simulink model "gm_soc_dvbs2_fpga"  (R2025b)
settings: Solver=VariableStepAuto  StartTime=0.0  StopTime=10.0  RelTol=1e-3
InitFcn:
  | soc_dvbs2_init;
undefined symbols (not defined in the file or in its folder): Add, coefficientsLog, coefficientsSqrt1, coefficientsSqrt2, dataBits, Deinterleaver, designMultirateFIR, noisePow, Shift, Short, soc_dvbs2_designFIRFilter, soc_dvbs2_txPacketBits, syncWord, txDataOut, txFiltCoeff, XData
libraries: simulink x304, hdlsllib x265, dspsigops x15, dsphdlfiltering2 x8, hdlmdlgenlib x6, dsphdlsigops2 x5, commseqgen3 x5, dsphdlmathfun2 x3, hwlogicconnlib x2, whdledac x2, commhdlcrc x2, whdlutilities x1
(part 15 of 36)

== system gm_soc_dvbs2_fpga/DVBS2/DVBS2 TxRx/Channel/AWGN Generator/Unit Variance Gaussian Noise/TausUniformRandGen/TausURNG2 ==
  note: S1
  note: S1
  note: S0
  Bit Shift : hdlsllib/Logic and Bit Operations/Bit Shift  mode=Shift Left Logical  N=double(13)
  Bit Shift1 : hdlsllib/Logic and Bit Operations/Bit Shift  mode=Shift Right Logical  N=double(19)
  Bit Shift2 : hdlsllib/Logic and Bit Operations/Bit Shift  mode=Shift Left Logical  N=double(12)
  Bit Shift3 : hdlsllib/Logic and Bit Operations/Bit Shift  mode=Shift Left Logical  N=double(2)
  Bit Shift4 : hdlsllib/Logic and Bit Operations/Bit Shift  mode=Shift Left Logical  N=double(4)
  Bit Shift5 : hdlsllib/Logic and Bit Operations/Bit Shift  mode=Shift Right Logical  N=double(25)
  Bit Shift6 : hdlsllib/Logic and Bit Operations/Bit Shift  mode=Shift Left Logical  N=double(3)
  Bit Shift7 : hdlsllib/Logic and Bit Operations/Bit Shift  mode=Shift Left Logical  N=double(17)
  Bit Shift8 : hdlsllib/Logic and Bit Operations/Bit Shift  mode=Shift Right Logical  N=double(11)
  Bitwise Operator{,2..3,5..6,8} (6 alike) : simulink/Logic and Bit Operations/Bitwise Operator  logicop=XOR  UseBitMask=off  NumInputPorts=2  BitMask=double(0)  BitMaskRealWorld=Real World Value
  Bitwise Operator1 : simulink/Logic and Bit Operations/Bitwise Operator  logicop=AND  UseBitMask=on  BitMask="fi(0,0,32,0,\"hex\",\"fffffffe\")"  BitMaskRealWorld=Real World Value
  Bitwise Operator4 : simulink/Logic and Bit Operations/Bitwise Operator  logicop=AND  UseBitMask=on  BitMask="fi(0,0,32,0,\"hex\",\"fffffff8\")"  BitMaskRealWorld=Real World Value
  Bitwise Operator7 : simulink/Logic and Bit Operations/Bitwise Operator  logicop=AND  UseBitMask=on  BitMask="fi(0,0,32,0,\"hex\",\"fffffff0\")"  BitMaskRealWorld=Real World Value
  Bitwise Operator9 : simulink/Logic and Bit Operations/Bitwise Operator  logicop=XOR  UseBitMask=off  NumInputPorts=3  BitMask=double(0)  BitMaskRealWorld=Real World Value
  Data Type Conversion : DataTypeConversion  OutDataTypeStr=fixdt('uint32')
  Data Type Conversion1 : DataTypeConversion  OutDataTypeStr=fixdt('uint32')
  Data Type Conversion2 : DataTypeConversion  OutDataTypeStr=fixdt('uint32')
  Delay : Delay  DelayLength=double(1)  InitialCondition=2343  SampleTime=6.25e-08
  Delay1 : Delay  DelayLength=double(1)  InitialCondition=323  SampleTime=6.25e-08
  Delay2 : Delay  DelayLength=double(1)  InitialCondition=833  SampleTime=6.25e-08
  b : Outport  SampleTime=6.25e-08
  wires:
  Bit Shift8/1 -> Bitwise Operator8/1
  Data Type Conversion/1 -> Bitwise Operator1/1, Bitwise Operator/2, Bit Shift/1
  Bitwise Operator8/1 -> Delay2/1, Bitwise Operator9/3
  Delay/1 -> Data Type Conversion/1
  Data Type Conversion1/1 -> Bitwise Operator4/1, Bit Shift3/1, Bitwise Operator3/2
  Bit Shift4/1 -> Bitwise Operator5/2
  Delay1/1 -> Data Type Conversion1/1
  Data Type Conversion2/1 -> Bitwise Operator6/2, Bitwise Operator7/1, Bit Shift6/1
  Bit Shift7/1 -> Bitwise Operator8/2
  Delay2/1 -> Data Type Conversion2/1
  Bit Shift/1 -> Bitwise Operator/1
  Bit Shift3/1 -> Bitwise Operator3/1
  Bitwise Operator4/1 -> Bit Shift4/1
  Bit Shift6/1 -> Bitwise Operator6/1
  Bitwise Operator7/1 -> Bit Shift7/1
  Bitwise Operator/1 -> Bit Shift1/1
  Bitwise Operator1/1 -> Bit Shift2/1
  Bitwise Operator3/1 -> Bit Shift5/1
  Bitwise Operator6/1 -> Bit Shift8/1
  Bit Shift1/1 -> Bitwise Operator2/1
  Bit Shift2/1 -> Bitwise Operator2/2
  Bit Shift5/1 -> Bitwise Operator5/1
  Bitwise Operator2/1 -> Delay/1, Bitwise Operator9/1
  Bitwise Operator5/1 -> Delay1/1, Bitwise Operator9/2
  Bitwise Operator9/1 -> b/1

== system gm_soc_dvbs2_fpga/DVBS2/DVBS2 TxRx/Channel/AWGN Generator/Unit Variance Gaussian Noise/logImplementation/log ==
  u0(48,48) : Inport  OutDataTypeStr=fixdt(0, 48, 48)  PortDimensions=1  SampleTime=6.25e-08
  FunctionEvaluation : Subsystem
  RangeReconstruction : Subsystem
  RangeReduction : Subsystem
  e : Outport  SampleTime=6.25e-08  VectorParamsAs1DForOutWhenUnconnected=off
  wires:
  FunctionEvaluation/2(exp_eOut) -> RangeReconstruction/2(exp_e)
  u0(48,48)/1 -> RangeReduction/1(x)
  RangeReduction/2(exp_e) -> FunctionEvaluation/2(exp_eIn)
  RangeReduction/1(x_e) -> FunctionEvaluation/1(x_e)
  FunctionEvaluation/1(y_e) -> RangeReconstruction/1(y_e)
  RangeReconstruction/1(e) -> e/1

== system gm_soc_dvbs2_fpga/DVBS2/DVBS2 TxRx/DVB-S2 HDL Receiver/Demod Deinterleave and FECDecode/DVBS2 HDL Deinterleaver/RAM/Single RAM Using Two RAMs ==
  wr_din : Inport  OutDataTypeStr=fixdt(1, 8, 4)  PortDimensions=1  SampleTime=7.8125e-09
  wr_addr : Inport  Port=2  OutDataTypeStr=fixdt(0, 17, 0)  PortDimensions=1  SampleTime=7.8125e-09
  wr_en : Inport  Port=3  OutDataTypeStr=boolean  PortDimensions=1  SampleTime=7.8125e-09
  rd_addr : Inport  Port=4  OutDataTypeStr=fixdt(0, 17, 0)  PortDimensions=1  SampleTime=7.8125e-09
  Delay : Delay  DelayLength=1
  Extract Bits : simulink/Logic and Bit Operations/Extract Bits  bitsToExtract=Range of bits  numBits=8  bitIdxRange=[0 15]  outScalingMode=Treat bit field as an integer
  Extract Bits1 : simulink/Logic and Bit Operations/Extract Bits  bitsToExtract=Range of bits  numBits=8  bitIdxRange=16  outScalingMode=Treat bit field as an integer
  Extract Bits2 : simulink/Logic and Bit Operations/Extract Bits  bitsToExtract=Range of bits  numBits=8  bitIdxRange=[0 15]  outScalingMode=Treat bit field as an integer
  Extract Bits3 : simulink/Logic and Bit Operations/Extract Bits  bitsToExtract=Range of bits  numBits=8  bitIdxRange=16  outScalingMode=Treat bit field as an integer
  Logical Operator1 : Logic  Operator=NOT  AllPortsSameDT=off  OutDataTypeStr=boolean
  Logical Operator2 : Logic  AllPortsSameDT=off  OutDataTypeStr=boolean
  Logical Operator3 : Logic  AllPortsSameDT=off  OutDataTypeStr=boolean
  Multiport Switch : MultiPortSwitch  DataPortOrder=Zero-based contiguous  Inputs=2  zeroidx=on  OutDataTypeStr=fixdt(1, 8, 4)  SaturateOnIntegerOverflow=off  InputSameDT=off
  Simple Dual Port RAM : hdlsllib/HDL RAMs/Simple Dual Port RAM  ram_size=nextpow2(ConfigRx.RAMCapacity/2)
  Simple Dual Port RAM1 : hdlsllib/HDL RAMs/Simple Dual Port RAM  ram_size=nextpow2(ConfigRx.RAMCapacity/2)
  rd_dout : Outport  SampleTime=7.8125e-09
  wires:
  wr_din/1 -> Simple Dual Port RAM/1, Simple Dual Port RAM1/1
  wr_addr/1 -> Extract Bits/1, Extract Bits1/1
  Extract Bits1/1 -> Logical Operator2/1, Logical Operator1/1
  Simple Dual Port RAM/1 -> Multiport Switch/2
  Logical Operator1/1 -> Logical Operator3/1
  Logical Operator3/1 -> Simple Dual Port RAM/3
  Extract Bits3/1 -> Delay/1
  wr_en/1 -> Logical Operator3/2, Logical Operator2/2
  rd_addr/1 -> Extract Bits3/1, Extract Bits2/1
  Extract Bits/1 -> Simple Dual Port RAM/2, Simple Dual Port RAM1/2
  Extract Bits2/1 -> Simple Dual Port RAM/4, Simple Dual Port RAM1/4
  Logical Operator2/1 -> Simple Dual Port RAM1/3
  Delay/1 -> Multiport Switch/1
  Simple Dual Port RAM1/1 -> Multiport Switch/3
  Multiport Switch/1 -> rd_dout/1

== system gm_soc_dvbs2_fpga/DVBS2/DVBS2 TxRx/DVB-S2 HDL Receiver/Demod Deinterleave and FECDecode/DVBS2 HDL Deinterleaver/RAM/Wrap Address ==
  u : Inport  OutDataTypeStr=fixdt(0, 18, 0)  PortDimensions=1  SampleTime=7.8125e-09
  Add : Sum  Inputs=+-  OutDataTypeStr=fixdt(0, 18, 0)
  Compare To Constant : simulink/Logic and Bit Operations/Compare To Constant  relop=>=  const=ConfigRx.RAMCapacity  OutDataTypeStr=boolean
  Constant : Constant  Value=ConfigRx.RAMCapacity  OutDataTypeStr=fixdt(0, 18, 0)  SampleTime=Tsamp
  Constant1 : Constant  Value=0  OutDataTypeStr=fixdt(0, 18, 0)  SampleTime=Tsamp
  Data Type Conversion : DataTypeConversion  OutDataTypeStr=fixdt(0,nextpow2(ConfigRx.RAMCapacity),0)  SaturateOnIntegerOverflow=off  RndMeth=Floor
  Switch : Switch  Criteria=u2 ~= 0  OutDataTypeStr=fixdt(0, 18, 0)  SaturateOnIntegerOverflow=off  InputSameDT=off
  Switch1 : Switch  Criteria=u2 ~= 0  OutDataTypeStr=fixdt(0, 18, 0)  SaturateOnIntegerOverflow=off  InputSameDT=off
  y : Outport  SampleTime=7.8125e-09
  wires:
  Add/1 -> Switch/1
  Constant1/1 -> Switch1/3
  Constant/1 -> Switch1/1
  u/1 -> Switch/3, Add/1, Compare To Constant/1
  Data Type Conversion/1 -> y/1
  Switch/1 -> Data Type Conversion/1
  Switch1/1 -> Add/2
  Compare To Constant/1 -> Switch/2, Switch1/2

== system gm_soc_dvbs2_fpga/DVBS2/DVBS2 TxRx/DVB-S2 HDL Receiver/Demod Deinterleave and FECDecode/DVBS2 HDL Deinterleaver/RAM Address Generator/Generate and Add Read Base Address ==
  readAddrIn : Inport  OutDataTypeStr=fixdt(0, 17, 0)  PortDimensions=1  SampleTime=7.8125e-09
  readValidIn : Inport  Port=2  OutDataTypeStr=boolean  PortDimensions=1  SampleTime=7.8125e-09
  startIn : Inport  Port=3  OutDataTypeStr=boolean  PortDimensions=1  SampleTime=7.8125e-09
  endIn : Inport  Port=4  OutDataTypeStr=boolean  PortDimensions=1  SampleTime=7.8125e-09
  Add : Sum  Inputs=|++  OutDataTypeStr=fixdt(0, 18, 0)
  Delay{,1,3..4,18} (5 alike) : Delay  DelayLength=1
  Delay{5..9,11,13..16,19..20} (12 alike) : Delay
  Gain : Gain  Gain=ConfigRx.ShortFrameLen  ParamDataTypeStr=fixdt(0,nextpow2(16200),0)  OutDataTypeStr=fixdt(0, 17, 0)
  HDL Counter : hdlsllib/Sources/HDL Counter  CountType=Count limited  CountInit=0  CountStep=1  CountMax=(ConfigRx.RAMCapacity/ConfigRx.ShortFrameLen) - 1  CountFromType=Initial value  CountFrom=0  CountResetPort=off  CountLoadPort=off  CountEnbPort=on  CountDirPort=off  CountHitOutputPort=off  CountDataType=Unsigned  CountWordLen=nextpow2((ConfigRx.RAMCapacity/ConfigRx.ShortFrameLen) - 1)  CountFracLen=0  CountSampTime=1
  Indicate End of Every ShortFrame Length Samples : Subsystem
  Logical Operator : Logic  AllPortsSameDT=off  OutDataTypeStr=boolean
  Unit Delay Enabled Synchronous3 : hdlsllib/Discrete/Unit Delay Enabled Synchronous  InitialCondition=0.0  SampleTime=-1
  readAddrOut : Outport  SampleTime=7.8125e-09
  readValidOut : Outport  Port=2  SampleTime=7.8125e-09
  readStartOut : Outport  Port=3  SampleTime=7.8125e-09
  readEndOut : Outport  Port=4  SampleTime=7.8125e-09
  wires:
  readValidIn/1 -> Logical Operator/2, Delay4/1
  Logical Operator/1 -> HDL Counter/1
  readAddrIn/1 -> Delay3/1, Indicate End of Every ShortFrame Length Samples/1(readAddr)
  startIn/1 -> Delay18/1
  Delay19/1 -> Delay20/1
  Delay18/1 -> Delay19/1
  Indicate End of Every ShortFrame Length Samples/1(endIndicate) -> Logical Operator/1
  Delay3/1 -> Delay13/1
  Delay4/1 -> Delay14/1
  Delay13/1 -> Delay15/1
  Gain/1 -> Delay6/1
  Delay20/1 -> readStartOut/1
  HDL Counter/1 -> Delay5/1
  Delay14/1 -> Delay16/1
  endIn/1 -> Delay1/1, Delay/1
  Delay5/1 -> Gain/1
  Delay16/1 -> readValidOut/1
  Delay15/1 -> Add/1
  Delay/1 -> Delay7/1
  Delay1/1 -> Delay9/1
  Delay7/1 -> Delay8/1
  Delay9/1 -> Delay11/1
  Delay6/1 -> Unit Delay Enabled Synchronous3/1
  Delay8/1 -> Unit Delay Enabled Synchronous3/2
  Delay11/1 -> readEndOut/1
  Unit Delay Enabled Synchronous3/1 -> Add/2
  Add/1 -> readAddrOut/1

== system gm_soc_dvbs2_fpga/DVBS2/DVBS2 TxRx/DVB-S2 HDL Receiver/Demod Deinterleave and FECDecode/DVBS2 HDL Deinterleaver/RAM Address Generator/Parameter Store FIFO ==
  writeVal : Inport  OutDataTypeStr=boolean  PortDimensions=1  SampleTime=7.8125e-09
  codIdxOut : Inport  Port=2  OutDataTypeStr=fixdt(0, 4, 0)  PortDimensions=1  SampleTime=7.8125e-09
  fecFrameOut : Inport  Port=3  OutDataTypeStr=boolean  PortDimensions=1  SampleTime=7.8125e-09
  readVal : Inport  Port=4  OutDataTypeStr=boolean  PortDimensions=1  SampleTime=7.8125e-09
  Delay1 : Delay  DelayLength=3
  Delay{6,8..14} (8 alike) : Delay  DelayLength=1
  Delay{3..5,7,15..20} (10 alike) : Delay
  Delay2 : Delay  DelayLength=3
  Fec Frame FIFO : hdlsllib/HDL RAMs/Simple Dual Port RAM  ram_size=log2(8)
  ReadVal Address : hdlsllib/Sources/HDL Counter  CountType=Count limited  CountInit=0  CountStep=1  CountMax=7  CountFromType=Initial value  CountFrom=0  CountResetPort=off  CountLoadPort=off  CountEnbPort=on  CountDirPort=off  CountHitOutputPort=off  CountDataType=Unsigned  CountWordLen=3  CountFracLen=0  CountSampTime=1
  WriteVal Address : hdlsllib/Sources/HDL Counter  CountType=Count limited  CountInit=0  CountStep=1  CountMax=7  CountFromType=Initial value  CountFrom=0  CountResetPort=off  CountLoadPort=off  CountEnbPort=on  CountDirPort=off  CountHitOutputPort=off  CountDataType=Unsigned  CountWordLen=3  CountFracLen=0  CountSampTime=1
  cod Idx FIFO : hdlsllib/HDL RAMs/Simple Dual Port RAM  ram_size=log2(8)
  codIdx : Outport  SampleTime=7.8125e-09
  fecframe : Outport  Port=2  SampleTime=7.8125e-09
  wires:
  writeVal/1 -> Delay9/1, Delay13/1, WriteVal Address/1
  readVal/1 -> ReadVal Address/1
  Delay1/1 -> codIdx/1
  codIdxOut/1 -> Delay6/1
  Delay13/1 -> Delay19/1
  Delay10/1 -> Delay16/1
  fecFrameOut/1 -> Delay11/1
  WriteVal Address/1 -> Delay12/1, Delay8/1
  ReadVal Address/1 -> Delay14/1, Delay10/1
  Delay9/1 -> Delay15/1
  Delay11/1 -> Delay17/1
  Delay12/1 -> Delay18/1
  Delay3/1 -> Delay1/1
  cod Idx FIFO/1 -> Delay3/1
  Delay14/1 -> Delay20/1
  Delay6/1 -> Delay5/1
  Delay8/1 -> Delay7/1
  Delay4/1 -> Delay2/1
  Delay15/1 -> cod Idx FIFO/3
  Delay17/1 -> Fec Frame FIFO/1
  Delay18/1 -> Fec Frame FIFO/2
  Delay19/1 -> Fec Frame FIFO/3
  Delay20/1 -> Fec Frame FIFO/4
  Delay16/1 -> cod Idx FIFO/4
  Delay5/1 -> cod Idx FIFO/1
  Delay7/1 -> cod Idx FIFO/2
  Fec Frame FIFO/1 -> Delay4/1
  Delay2/1 -> fecframe/1

== system gm_soc_dvbs2_fpga/DVBS2/DVBS2 TxRx/DVB-S2 HDL Receiver/Demod Deinterleave and FECDecode/DVBS2 HDL Deinterleaver/RAM Address Generator/Read Offset Address ==
  maxR : Inport  OutDataTypeStr=uint16  PortDimensions=1  SampleTime=7.8125e-09
  maxC : Inport  Port=2  OutDataTypeStr=fixdt(0, 3, 0)  PortDimensions=1  SampleTime=7.8125e-09
  modcodIs12 : Inport  Port=3  OutDataTypeStr=boolean  PortDimensions=1  SampleTime=7.8125e-09
  wrAddr : Inport  Port=4  OutDataTypeStr=uint16  PortDimensions=1  SampleTime=7.8125e-09
  wrEnb : Inport  Port=5  OutDataTypeStr=boolean  PortDimensions=1  SampleTime=7.8125e-09
  Compute Read Offset Address : Subsystem
  Delay{,1..6,9} (8 alike) : Delay  DelayLength=4
  Generate Signal for End of Frame : Subsystem
  Read Offset Address Signals Generator : Subsystem
  Read Offset Address Signals Generator_term3 : Terminator
  readAddr : Outport  SampleTime=7.8125e-09
  readValid : Outport  Port=2  SampleTime=7.8125e-09
  startOut : Outport  Port=3  SampleTime=7.8125e-09
  endOut : Outport  Port=4  SampleTime=7.8125e-09
  wires:
  wrEnb/1 -> Delay4/1
  wrAddr/1 -> Delay3/1
  modcodIs12/1 -> Delay2/1
  maxC/1 -> Delay1/1, Generate Signal for End of Frame/2(maxC)
  maxR/1 -> Delay/1, Generate Signal for End of Frame/1(maxR)
  Delay6/1 -> startOut/1
  Delay1/1 -> Read Offset Address Signals Generator/3(maxC)
  Delay5/1 -> endOut/1
  Delay/1 -> Read Offset Address Signals Generator/1(maxR)
  Generate Signal for End of Frame/1(chkwrAddrEnd) -> Read Offset Address Signals Generator/2(chkwrAddrEnd)
  Delay2/1 -> Read Offset Address Signals Generator/4(modcodIs12)
  Delay3/1 -> Read Offset Address Signals Generator/5(wrAddr)
  Delay4/1 -> Read Offset Address Signals Generator/6(wrEnb)
  Read Offset Address Signals Generator/1(curCorROut) -> Compute Read Offset Address/1(curR)
  Read Offset Address Signals Generator/2(maxRorCOut) -> Compute Read Offset Address/2(maxC)
  Read Offset Address Signals Generator/3(curRorCOut) -> Compute Read Offset Address/3(curC)
  Read Offset Address Signals Generator/4(modcodIs12Out) -> Read Offset Address Signals Generator_term3/1
  Read Offset Address Signals Generator/5(startOut) -> Delay6/1
  Read Offset Address Signals Generator/6(endOut) -> Delay5/1
  Read Offset Address Signals Generator/7(readValid) -> Delay9/1
  Delay9/1 -> readValid/1
  Compute Read Offset Address/1(addr) -> readAddr/1

== system gm_soc_dvbs2_fpga/DVBS2/DVBS2 TxRx/DVB-S2 HDL Receiver/Demod Deinterleave and FECDecode/DVBS2 HDL Deinterleaver/RAM Address Generator/Write Offset Address ==
  fecframe : Inport  OutDataTypeStr=boolean  PortDimensions=1  SampleTime=7.8125e-09
  enb : Inport  Port=2  OutDataTypeStr=boolean  PortDimensions=1  SampleTime=7.8125e-09
  Compare To Constant : simulink/Logic and Bit Operations/Compare To Constant  relop===  const=ConfigRx.ShortFrameLen - 1  OutDataTypeStr=boolean
  Data Type Conversion : DataTypeConversion  OutDataTypeStr=uint16  SaturateOnIntegerOverflow=off  RndMeth=Floor
  Delay{1..12} (12 alike) : Delay  DelayLength=1
  Logical Operator : Logic  Inputs=3  AllPortsSameDT=off  OutDataTypeStr=boolean
  Switch : Switch  Criteria=u2 ~= 0  OutDataTypeStr=uint16  SaturateOnIntegerOverflow=off  InputSameDT=off
  Write Offset Address Normal Frame : hdlsllib/Sources/HDL Counter  CountType=Count limited  CountInit=0  CountStep=1  CountMax=ConfigRx.NormalFrameLen - 1  CountFromType=Initial value  CountFrom=0  CountResetPort=on  CountLoadPort=off  CountEnbPort=on  CountDirPort=off  CountHitOutputPort=off  CountDataType=Unsigned  CountWordLen=nextpow2(ConfigRx.NormalFrameLen - 1)  CountFracLen=0  CountSampTime=1
  Write Offset Address Short Frame : hdlsllib/Sources/HDL Counter  CountType=Count limited  CountInit=0  CountStep=1  CountMax=ConfigRx.ShortFrameLen - 1  CountFromType=Initial value  CountFrom=0  CountResetPort=off  CountLoadPort=off  CountEnbPort=on  CountDirPort=off  CountHitOutputPort=off  CountDataType=Unsigned  CountWordLen=nextpow2(ConfigRx.ShortFrameLen - 1)  CountFracLen=0  CountSampTime=1
  addr : Outport  SampleTime=7.8125e-09
  wires:
  fecframe/1 -> Delay12/1
  enb/1 -> Delay10/1
  Delay9/1 -> Delay7/1, Logical Operator/3
  Delay11/1 -> Logical Operator/1, Delay4/1
  Delay1/1 -> Switch/2
  Delay3/1 -> Data Type Conversion/1
  Delay12/1 -> Delay11/1
  Delay8/1 -> Compare To Constant/1, Delay3/1
  Delay4/1 -> Delay1/1
  Delay10/1 -> Delay9/1, Write Offset Address Short Frame/1
  Write Offset Address Short Frame/1 -> Delay8/1
  Switch/1 -> addr/1
  Compare To Constant/1 -> Logical Operator/2
  Data Type Conversion/1 -> Delay5/1
  Logical Operator/1 -> Delay6/1
  Delay6/1 -> Write Offset Address Normal Frame/1
  Delay2/1 -> Switch/3
  Delay7/1 -> Write Offset Address Normal Frame/2
  Write Offset Address Normal Frame/1 -> Delay2/1
  Delay5/1 -> Switch/1

== system gm_soc_dvbs2_fpga/DVBS2/DVBS2 TxRx/DVB-S2 HDL Receiver/Demod Deinterleave and FECDecode/DVBS2 HDL Deinterleaver/RAM Address Generator/nRows and nColumns ==
  captureIn : Inport  OutDataTypeStr=boolean  PortDimensions=1  SampleTime=7.8125e-09
  modIdx : Inport  Port=2  OutDataTypeStr=fixdt(0, 2, 0)  PortDimensions=1  SampleTime=7.8125e-09
  codIdx : Inport  Port=3  OutDataTypeStr=fixdt(0, 4, 0)  PortDimensions=1  SampleTime=7.8125e-09
  fecFrame : Inport  Port=4  OutDataTypeStr=boolean  PortDimensions=1  SampleTime=7.8125e-09
  Compare To Constant : simulink/Logic and Bit Operations/Compare To Constant  relop===  const="fi(0,0,2,0,\"hex\",\"1\")"  OutDataTypeStr=boolean
  Compare To Constant1 : simulink/Logic and Bit Operations/Compare To Constant  relop===  const="fi(0,0,4,0,\"hex\",\"4\")"  OutDataTypeStr=boolean
  Data Type Conversion : DataTypeConversion  OutDataTypeStr=uint16  SampleTime=7.8125e-09  SaturateOnIntegerOverflow=off  RndMeth=Floor
  Delay{1..14} (14 alike) : Delay  DelayLength=double(2)  InitialCondition=0  SampleTime=7.8125e-09
  Logical Operator : Logic  AllPortsSameDT=off  OutDataTypeStr=boolean  SampleTime=7.8125e-09
  MaxC LUT : Lookup_n-D  NumberOfTableDimensions=1  BreakpointsSpecification=Even spacing  BreakpointsForDimension1=[-5:5]  BreakpointsForDimension1FirstPoint=0  Table=[1 3 4 5]  TableDataTypeStr=fixdt(0,3,0)  InterpMethod=Flat  InternalRulePriority=Speed  OutDataTypeStr=fixdt(0,3,0)  RndMeth=Simplest
  MaxR Normal LUT : Lookup_n-D  NumberOfTableDimensions=1  BreakpointsSpecification=Even spacing  BreakpointsForDimension1=[-5:5]  BreakpointsForDimension1FirstPoint=0  Table=64800./[1 3 4 5]  TableDataTypeStr=fixdt(0,nextpow2(64800),0)  InterpMethod=Flat  InternalRulePriority=Speed  OutDataTypeStr=fixdt(0,nextpow2(64800),0)  RndMeth=Simplest
  MaxR Short LUT : Lookup_n-D  NumberOfTableDimensions=1  BreakpointsSpecification=Even spacing  BreakpointsForDimension1=[-5:5]  BreakpointsForDimension1FirstPoint=0  Table=16200./[1 3 4 5]  TableDataTypeStr=fixdt(0,nextpow2(16200),0)  InterpMethod=Flat  InternalRulePriority=Speed  OutDataTypeStr=fixdt(0,nextpow2(16200),0)  RndMeth=Simplest
  maxR_switch : MultiPortSwitch  DataPortOrder=Zero-based contiguous  Inputs=2  DiagnosticForDefault=None  zeroidx=on  OutDataTypeStr=uint16  SampleTime=7.8125e-09  SaturateOnIntegerOverflow=off  InputSameDT=off
  captureOut : Outport  SampleTime=7.8125e-09
  codIdxOut : Outport  Port=2  SampleTime=7.8125e-09
  fecFrameOut : Outport  Port=3  SampleTime=7.8125e-09
  maxR : Outport  Port=4  SampleTime=7.8125e-09
  maxC : Outport  Port=5  SampleTime=7.8125e-09
  isMODOCD12 : Outport  Port=6  SampleTime=7.8125e-09
  wires:
  captureIn/1 -> Delay2/1
  modIdx/1 -> Delay9/1, Delay11/1, Delay5/1, Delay10/1
  codIdx/1 -> Delay6/1
  Delay10/1 -> MaxR Short LUT/1
  Delay11/1 -> MaxC LUT/1
  Delay14/1 -> maxR_switch/2
  Delay9/1 -> MaxR Normal LUT/1
  Delay6/1 -> Delay8/1
  Delay5/1 -> Delay7/1
  MaxC LUT/1 -> Delay12/1
  Delay2/1 -> Delay4/1
  fecFrame/1 -> Delay1/1
  Delay7/1 -> Compare To Constant/1
  Delay8/1 -> Compare To Constant1/1, codIdxOut/1
  Delay3/1 -> maxR_switch/1, fecFrameOut/1
  MaxR Normal LUT/1 -> Delay14/1
  MaxR Short LUT/1 -> Delay13/1
  Delay4/1 -> captureOut/1
  Delay12/1 -> maxC/1
  Delay1/1 -> Delay3/1
  Compare To Constant1/1 -> Logical Operator/2
  Compare To Constant/1 -> Logical Operator/1
  Delay13/1 -> Data Type Conversion/1
  Logical Operator/1 -> isMODOCD12/1
  Data Type Conversion/1 -> maxR_switch/3
  maxR_switch/1 -> maxR/1

== system gm_soc_dvbs2_fpga/DVBS2/DVBS2 TxRx/DVB-S2 HDL Receiver/Stream Recovery/BB Decoder/Extract BBHeader/Extract DFL ==
  bitsIn : Inport  OutDataTypeStr=boolean  PortDimensions=1  SampleTime=7.8125e-09
  idx : Inport  Port=2  OutDataTypeStr=fixdt(0, 7, 0)  PortDimensions=1  SampleTime=7.8125e-09
  validIn : Inport  Port=3  OutDataTypeStr=boolean  PortDimensions=1  SampleTime=7.8125e-09
  Add : Sum  OutDataTypeStr=uint16  AccumDataTypeStr=uint16  SampleTime=7.8125e-09
  Compare To Constant : simulink/Logic and Bit Operations/Compare To Constant  relop=>=  const="fi(0,0,7,0,\"hex\",\"20\")"  OutDataTypeStr=boolean
  Compare To Constant1 : simulink/Logic and Bit Operations/Compare To Constant  relop=<=  const="fi(0,0,7,0,\"hex\",\"2f\")"  OutDataTypeStr=boolean
  Compare To Constant2 : simulink/Logic and Bit Operations/Compare To Constant  relop===  const="fi(0,0,7,0,\"hex\",\"30\")"  OutDataTypeStr=boolean
  Data Type Conversion : DataTypeConversion  OutDataTypeStr=uint16  SampleTime=7.8125e-09  SaturateOnIntegerOverflow=off  RndMeth=Floor
  Gain : Gain  Gain="fi(0,0,2,0,\"hex\",\"2\")"  ParamDataTypeStr=fixdt(0, 2, 0)  OutDataTypeStr=uint16  SampleTime=7.8125e-09
  Logical Operator : Logic  Inputs=3  AllPortsSameDT=off  OutDataTypeStr=boolean  SampleTime=7.8125e-09
  Logical Operator1 : Logic  AllPortsSameDT=off  OutDataTypeStr=boolean  SampleTime=7.8125e-09
  Unit Delay Enabled Resettable Synchronous : hdlsllib/Discrete/Unit Delay Enabled Resettable Synchronous  InitialCondition=double(0)  SampleTime=-1
  Unit Delay Enabled Synchronous : hdlsllib/Discrete/Unit Delay Enabled Synchronous  InitialCondition=double(0)  SampleTime=-1
  DFL : Outport  SampleTime=7.8125e-09
  wires:
  idx/1 -> Compare To Constant1/1, Compare To Constant2/1, Compare To Constant/1
  Unit Delay Enabled Synchronous/1 -> DFL/1
  Compare To Constant/1 -> Logical Operator/1
  Compare To Constant1/1 -> Logical Operator/2
  Compare To Constant2/1 -> Logical Operator1/1
  bitsIn/1 -> Data Type Conversion/1
  validIn/1 -> Logical Operator1/2, Logical Operator/3
  Unit Delay Enabled Resettable Synchronous/1 -> Unit Delay Enabled Synchronous/1, Gain/1
  Logical Operator/1 -> Unit Delay Enabled Resettable Synchronous/2
  Logical Operator1/1 -> Unit Delay Enabled Synchronous/2, Unit Delay Enabled Resettable Synchronous/3
  Add/1 -> Unit Delay Enabled Resettable Synchronous/1
  Data Type Conversion/1 -> Add/1
  Gain/1 -> Add/2

== system gm_soc_dvbs2_fpga/DVBS2/DVBS2 TxRx/DVB-S2 HDL Receiver/Stream Recovery/BB Decoder/Extract BBHeader/Extract MATYPE1 ==
  bitsIn : Inport  OutDataTypeStr=boolean  PortDimensions=1  SampleTime=7.8125e-09
  idx : Inport  Port=2  OutDataTypeStr=fixdt(0, 7, 0)  PortDimensions=1  SampleTime=7.8125e-09
  validIn : Inport  Port=3  OutDataTypeStr=boolean  PortDimensions=1  SampleTime=7.8125e-09
  Bit Concat : hdlsllib/Logic and Bit Operations/Bit Concat  numInputs=2
  Bit Concat1 : hdlsllib/Logic and Bit Operations/Bit Concat  numInputs=2
  Compare To Constant : simulink/Logic and Bit Operations/Compare To Constant  relop===  const=0  OutDataTypeStr=boolean
  Compare To Constant1 : simulink/Logic and Bit Operations/Compare To Constant  relop===  const=1  OutDataTypeStr=boolean
  Compare To Constant2 : simulink/Logic and Bit Operations/Compare To Constant  relop===  const=2  OutDataTypeStr=boolean
  Compare To Constant3 : simulink/Logic and Bit Operations/Compare To Constant  relop===  const=3  OutDataTypeStr=boolean
  Compare To Constant4 : simulink/Logic and Bit Operations/Compare To Constant  relop===  const=4  OutDataTypeStr=boolean
  Compare To Constant5 : simulink/Logic and Bit Operations/Compare To Constant  relop===  const=5  OutDataTypeStr=boolean
  Compare To Constant6 : simulink/Logic and Bit Operations/Compare To Constant  relop===  const=6  OutDataTypeStr=boolean
  Compare To Constant7 : simulink/Logic and Bit Operations/Compare To Constant  relop===  const=7  OutDataTypeStr=boolean
  Delay{,1..6} (7 alike) : Delay  DelayLength=1
  Logical Operator{,1..7} (8 alike) : Logic  AllPortsSameDT=off  OutDataTypeStr=boolean
  Unit Delay Enabled Synchronous{,1..7} (8 alike) : hdlsllib/Discrete/Unit Delay Enabled Synchronous  InitialCondition=0.0  SampleTime=-1
  TSorGS : Outport  SampleTime=7.8125e-09
  SISorMIS : Outport  Port=2  SampleTime=7.8125e-09
  CCMorACM : Outport  Port=3  SampleTime=7.8125e-09
  ISSYI : Outport  Port=4  SampleTime=7.8125e-09
  NPD : Outport  Port=5  SampleTime=7.8125e-09
  RO : Outport  Port=6  SampleTime=7.8125e-09
  wires:
  Unit Delay Enabled Synchronous4/1 -> ISSYI/1
  Compare To Constant6/1 -> Logical Operator6/1
  Compare To Constant7/1 -> Logical Operator7/1
  idx/1 -> Compare To Constant7/1, Compare To Constant3/1, Compare To Constant4/1, Compare To Constant2/1, Compare To Constant5/1, Compare To Constant1/1, Compare To Constant6/1, Compare To Constant/1
  Compare To Constant3/1 -> Logical Operator3/1
  Compare To Constant4/1 -> Logical Operator4/1
  Compare To Constant2/1 -> Logical Operator2/1
  Compare To Constant5/1 -> Logical Operator5/1
  Unit Delay Enabled Synchronous7/1 -> RO/1
  validIn/1 -> Logical Operator5/2, Logical Operator6/2, Logical Operator4/2, Logical Operator3/2, Logical Operator2/2, Logical Operator/2, Logical Operator1/2, Logical Operator7/2
  Bit Concat1/1 -> Unit Delay Enabled Synchronous7/1
  Compare To Constant1/1 -> Logical Operator1/1
  Compare To Constant/1 -> Logical Operator/1
  Logical Operator/1 -> Unit Delay Enabled Synchronous/2
  Logical Operator4/1 -> Delay4/1
  Logical Operator2/1 -> Delay2/1
  Logical Operator6/1 -> Unit Delay Enabled Synchronous6/2
  Logical Operator3/1 -> Delay3/1
  Logical Operator7/1 -> Delay6/1
  Logical Operator1/1 -> Delay/1
  Logical Operator5/1 -> Delay5/1
  bitsIn/1 -> Unit Delay Enabled Synchronous6/1, Unit Delay Enabled Synchronous/1, Delay1/1
  Delay4/1 -> Unit Delay Enabled Synchronous4/2
  Delay1/1 -> Bit Concat1/2, Unit Delay Enabled Synchronous3/1, Unit Delay Enabled Synchronous4/1, Unit Delay Enabled Synchronous5/1, Unit Delay Enabled Synchronous2/1, Bit Concat/2
  Unit Delay Enabled Synchronous6/1 -> Bit Concat1/1
  Delay2/1 -> Unit Delay Enabled Synchronous2/2
  Delay5/1 -> Unit Delay Enabled Synchronous5/2
  Unit Delay Enabled Synchronous/1 -> Bit Concat/1
  Delay3/1 -> Unit Delay Enabled Synchronous3/2
  Delay6/1 -> Unit Delay Enabled Synchronous7/2
  Unit Delay Enabled Synchronous2/1 -> SISorMIS/1
  Unit Delay Enabled Synchronous5/1 -> NPD/1
  Bit Concat/1 -> Unit Delay Enabled Synchronous1/1
  Delay/1 -> Unit Delay Enabled Synchronous1/2
  Unit Delay Enabled Synchronous3/1 -> CCMorACM/1
  Unit Delay Enabled Synchronous1/1 -> TSorGS/1

== system gm_soc_dvbs2_fpga/DVBS2/DVBS2 TxRx/DVB-S2 HDL Receiver/Stream Recovery/BB Decoder/Extract BBHeader/Extract MATYPE2 ==
  bitsIn : Inport  OutDataTypeStr=boolean  PortDimensions=1  SampleTime=7.8125e-09
  idx : Inport  Port=2  OutDataTypeStr=fixdt(0, 7, 0)  PortDimensions=1  SampleTime=7.8125e-09
  validIn : Inport  Port=3  OutDataTypeStr=boolean  PortDimensions=1  SampleTime=7.8125e-09
  Add : Sum  OutDataTypeStr=uint8  AccumDataTypeStr=uint8  SampleTime=7.8125e-09
  Compare To Constant : simulink/Logic and Bit Operations/Compare To Constant  relop=>=  const="fi(0,0,7,0,\"hex\",\"08\")"  OutDataTypeStr=boolean
  Compare To Constant1 : simulink/Logic and Bit Operations/Compare To Constant  relop=<=  const="fi(0,0,7,0,\"hex\",\"0f\")"  OutDataTypeStr=boolean
  Compare To Constant2 : simulink/Logic and Bit Operations/Compare To Constant  relop===  const="fi(0,0,7,0,\"hex\",\"10\")"  OutDataTypeStr=boolean
  Data Type Conversion : DataTypeConversion  OutDataTypeStr=uint8  SampleTime=7.8125e-09  SaturateOnIntegerOverflow=off  RndMeth=Floor
  Gain : Gain  Gain="fi(0,0,2,0,\"hex\",\"2\")"  ParamDataTypeStr=fixdt(0, 2, 0)  OutDataTypeStr=uint8  SampleTime=7.8125e-09
  Logical Operator : Logic  Inputs=3  AllPortsSameDT=off  OutDataTypeStr=boolean  SampleTime=7.8125e-09
  Logical Operator1 : Logic  AllPortsSameDT=off  OutDataTypeStr=boolean  SampleTime=7.8125e-09
  Unit Delay Enabled Resettable Synchronous : hdlsllib/Discrete/Unit Delay Enabled Resettable Synchronous  InitialCondition=double(0)  SampleTime=-1
  Unit Delay Enabled Synchronous : hdlsllib/Discrete/Unit Delay Enabled Synchronous  InitialCondition=double(0)  SampleTime=-1
  MIS_ISI : Outport  SampleTime=7.8125e-09
  wires:
  idx/1 -> Compare To Constant2/1, Compare To Constant1/1, Compare To Constant/1
  Compare To Constant/1 -> Logical Operator/1
  validIn/1 -> Logical Operator1/2, Logical Operator/3
  Compare To Constant1/1 -> Logical Operator/2
  Logical Operator/1 -> Unit Delay Enabled Resettable Synchronous/2
  Compare To Constant2/1 -> Logical Operator1/1
  Logical Operator1/1 -> Unit Delay Enabled Synchronous/2, Unit Delay Enabled Resettable Synchronous/3
  bitsIn/1 -> Data Type Conversion/1
  Unit Delay Enabled Resettable Synchronous/1 -> Unit Delay Enabled Synchronous/1, Gain/1
  Add/1 -> Unit Delay Enabled Resettable Synchronous/1
  Data Type Conversion/1 -> Add/1
  Gain/1 -> Add/2
  Unit Delay Enabled Synchronous/1 -> MIS_ISI/1

== system gm_soc_dvbs2_fpga/DVBS2/DVBS2 TxRx/DVB-S2 HDL Receiver/Stream Recovery/BB Decoder/Extract BBHeader/Extract SYNC ==
  bitsIn : Inport  OutDataTypeStr=boolean  PortDimensions=1  SampleTime=7.8125e-09
  idx : Inport  Port=2  OutDataTypeStr=fixdt(0, 7, 0)  PortDimensions=1  SampleTime=7.8125e-09
  validIn : Inport  Port=3  OutDataTypeStr=boolean  PortDimensions=1  SampleTime=7.8125e-09
  Add : Sum  OutDataTypeStr=uint8  AccumDataTypeStr=uint8  SampleTime=7.8125e-09
  Compare To Constant : simulink/Logic and Bit Operations/Compare To Constant  relop=>=  const="fi(0,0,7,0,\"hex\",\"30\")"  OutDataTypeStr=boolean
  Compare To Constant1 : simulink/Logic and Bit Operations/Compare To Constant  relop=<=  const="fi(0,0,7,0,\"hex\",\"37\")"  OutDataTypeStr=boolean
  Compare To Constant2 : simulink/Logic and Bit Operations/Compare To Constant  relop===  const="fi(0,0,7,0,\"hex\",\"38\")"  OutDataTypeStr=boolean
  Data Type Conversion : DataTypeConversion  OutDataTypeStr=uint8  SampleTime=7.8125e-09  SaturateOnIntegerOverflow=off  RndMeth=Floor
  Gain : Gain  Gain="fi(0,0,2,0,\"hex\",\"2\")"  ParamDataTypeStr=fixdt(0, 2, 0)  OutDataTypeStr=uint8  SampleTime=7.8125e-09
  Logical Operator : Logic  Inputs=3  AllPortsSameDT=off  OutDataTypeStr=boolean  SampleTime=7.8125e-09
  Logical Operator1 : Logic  AllPortsSameDT=off  OutDataTypeStr=boolean  SampleTime=7.8125e-09
  Unit Delay Enabled Resettable Synchronous : hdlsllib/Discrete/Unit Delay Enabled Resettable Synchronous  InitialCondition=double(0)  SampleTime=-1
  Unit Delay Enabled Synchronous : hdlsllib/Discrete/Unit Delay Enabled Synchronous  InitialCondition=double(0)  SampleTime=-1
  SYNC : Outport  SampleTime=7.8125e-09
  wires:
  idx/1 -> Compare To Constant2/1, Compare To Constant1/1, Compare To Constant/1
  Unit Delay Enabled Synchronous/1 -> SYNC/1
  Compare To Constant/1 -> Logical Operator/1
  Compare To Constant1/1 -> Logical Operator/2
  Compare To Constant2/1 -> Logical Operator1/1
  bitsIn/1 -> Data Type Conversion/1
  validIn/1 -> Logical Operator1/2, Logical Operator/3
  Unit Delay Enabled Resettable Synchronous/1 -> Unit Delay Enabled Synchronous/1, Gain/1
  Logical Operator/1 -> Unit Delay Enabled Resettable Synchronous/2
  Logical Operator1/1 -> Unit Delay Enabled Synchronous/2, Unit Delay Enabled Resettable Synchronous/3
  Add/1 -> Unit Delay Enabled Resettable Synchronous/1
  Data Type Conversion/1 -> Add/1
  Gain/1 -> Add/2

== system gm_soc_dvbs2_fpga/DVBS2/DVBS2 TxRx/DVB-S2 HDL Receiver/Stream Recovery/BB Decoder/Extract BBHeader/Extract SYNCD ==
  bitsIn : Inport  OutDataTypeStr=boolean  PortDimensions=1  SampleTime=7.8125e-09
  idx : Inport  Port=2  OutDataTypeStr=fixdt(0, 7, 0)  PortDimensions=1  SampleTime=7.8125e-09
  validIn : Inport  Port=3  OutDataTypeStr=boolean  PortDimensions=1  SampleTime=7.8125e-09
  Add : Sum  OutDataTypeStr=uint16  AccumDataTypeStr=uint16  SampleTime=7.8125e-09
  Compare To Constant : simulink/Logic and Bit Operations/Compare To Constant  relop=>=  const="fi(0,0,7,0,\"hex\",\"38\")"  OutDataTypeStr=boolean
  Compare To Constant1 : simulink/Logic and Bit Operations/Compare To Constant  relop=<=  const="fi(0,0,7,0,\"hex\",\"47\")"  OutDataTypeStr=boolean
  Data Type Conversion : DataTypeConversion  OutDataTypeStr=uint16  SampleTime=7.8125e-09  SaturateOnIntegerOverflow=off  RndMeth=Floor
  Delay : Delay  DelayLength=double(1)  InitialCondition=0  SampleTime=7.8125e-09
  Gain : Gain  Gain="fi(0,0,2,0,\"hex\",\"2\")"  ParamDataTypeStr=fixdt(0, 2, 0)  OutDataTypeStr=uint16  SampleTime=7.8125e-09
  Logical Operator : Logic  Inputs=3  AllPortsSameDT=off  OutDataTypeStr=boolean  SampleTime=7.8125e-09
  Logical Operator1 : Logic  AllPortsSameDT=off  OutDataTypeStr=boolean  SampleTime=7.8125e-09
  Unit Delay Enabled Resettable Synchronous : hdlsllib/Discrete/Unit Delay Enabled Resettable Synchronous  InitialCondition=double(0)  SampleTime=-1
  Unit Delay Enabled Synchronous : hdlsllib/Discrete/Unit Delay Enabled Synchronous  InitialCondition=double(0)  SampleTime=-1
  DFL : Outport  SampleTime=7.8125e-09
  wires:
  Delay/1 -> Unit Delay Enabled Synchronous/2, Unit Delay Enabled Resettable Synchronous/3
  idx/1 -> Compare To Constant1/1, Compare To Constant/1
  Logical Operator/1 -> Unit Delay Enabled Resettable Synchronous/2
  Compare To Constant/1 -> Logical Operator/1
  Compare To Constant1/1 -> Logical Operator1/1, Logical Operator/2
  validIn/1 -> Logical Operator1/2, Logical Operator/3
  Logical Operator1/1 -> Delay/1
  bitsIn/1 -> Data Type Conversion/1
  Unit Delay Enabled Resettable Synchronous/1 -> Unit Delay Enabled Synchronous/1, Gain/1
  Add/1 -> Unit Delay Enabled Resettable Synchronous/1
  Data Type Conversion/1 -> Add/1
  Gain/1 -> Add/2
  Unit Delay Enabled Synchronous/1 -> DFL/1

== system gm_soc_dvbs2_fpga/DVBS2/DVBS2 TxRx/DVB-S2 HDL Receiver/Stream Recovery/BB Decoder/Extract BBHeader/Extract UPL ==
  bitsIn : Inport  OutDataTypeStr=boolean  PortDimensions=1  SampleTime=7.8125e-09
  idx : Inport  Port=2  OutDataTypeStr=fixdt(0, 7, 0)  PortDimensions=1  SampleTime=7.8125e-09
  validIn : Inport  Port=3  OutDataTypeStr=boolean  PortDimensions=1  SampleTime=7.8125e-09
  Add : Sum  OutDataTypeStr=uint16  AccumDataTypeStr=uint16  SampleTime=7.8125e-09
  Compare To Constant : simulink/Logic and Bit Operations/Compare To Constant  relop=>=  const="fi(0,0,7,0,\"hex\",\"10\")"  OutDataTypeStr=boolean
  Compare To Constant1 : simulink/Logic and Bit Operations/Compare To Constant  relop=<=  const="fi(0,0,7,0,\"hex\",\"1f\")"  OutDataTypeStr=boolean
  Compare To Constant2 : simulink/Logic and Bit Operations/Compare To Constant  relop===  const="fi(0,0,7,0,\"hex\",\"20\")"  OutDataTypeStr=boolean
  Data Type Conversion : DataTypeConversion  OutDataTypeStr=uint16  SampleTime=7.8125e-09  SaturateOnIntegerOverflow=off  RndMeth=Floor
  Gain : Gain  Gain="fi(0,0,2,0,\"hex\",\"2\")"  ParamDataTypeStr=fixdt(0, 2, 0)  OutDataTypeStr=uint16  SampleTime=7.8125e-09
  Logical Operator : Logic  Inputs=3  AllPortsSameDT=off  OutDataTypeStr=boolean  SampleTime=7.8125e-09
  Logical Operator1 : Logic  AllPortsSameDT=off  OutDataTypeStr=boolean  SampleTime=7.8125e-09
  Unit Delay Enabled Resettable Synchronous : hdlsllib/Discrete/Unit Delay Enabled Resettable Synchronous  InitialCondition=double(0)  SampleTime=-1
  Unit Delay Enabled Synchronous : hdlsllib/Discrete/Unit Delay Enabled Synchronous  InitialCondition=double(0)  SampleTime=-1
  UPL : Outport  SampleTime=7.8125e-09
  wires:
  idx/1 -> Compare To Constant2/1, Compare To Constant/1, Compare To Constant1/1
  Unit Delay Enabled Synchronous/1 -> UPL/1
  Compare To Constant/1 -> Logical Operator/1
  Compare To Constant1/1 -> Logical Operator/2
  bitsIn/1 -> Data Type Conversion/1
  validIn/1 -> Logical Operator1/2, Logical Operator/3
  Logical Operator/1 -> Unit Delay Enabled Resettable Synchronous/2
  Compare To Constant2/1 -> Logical Operator1/1
  Logical Operator1/1 -> Unit Delay Enabled Synchronous/2, Unit Delay Enabled Resettable Synchronous/3
  Unit Delay Enabled Resettable Synchronous/1 -> Unit Delay Enabled Synchronous/1, Gain/1
  Add/1 -> Unit Delay Enabled Resettable Synchronous/1
  Data Type Conversion/1 -> Add/1
  Gain/1 -> Add/2

== system gm_soc_dvbs2_fpga/DVBS2/DVBS2 TxRx/DVB-S2 HDL Receiver/Stream Recovery/BB Decoder/Extract BBHeader/Saturate UPL value ==
  UPL : Inport  OutDataTypeStr=uint16  PortDimensions=1  SampleTime=7.8125e-09
  DFL : Inport  Port=2  OutDataTypeStr=uint16  PortDimensions=1  SampleTime=7.8125e-09
  Add : Sum  Inputs=+-  OutDataTypeStr=uint16
  Constant : Constant  Value=10  OutDataTypeStr=fixdt(0,4,0)  SampleTime=-1
  Relational Operator : RelationalOperator  Operator=>  OutDataTypeStr=boolean  RndMeth=Simplest  InputSameDT=off
  Switch : Switch  Criteria=u2 ~= 0  OutDataTypeStr=uint16  SaturateOnIntegerOverflow=off  InputSameDT=off
  saturatedUPL : Outport  SampleTime=7.8125e-09
  wires:
  Relational Operator/1 -> Switch/2
  Add/1 -> Switch/1, Relational Operator/2
  Constant/1 -> Add/2
  DFL/1 -> Add/1
  Switch/1 -> saturatedUPL/1
  UPL/1 -> Switch/3, Relational Operator/1

== system gm_soc_dvbs2_fpga/DVBS2/DVBS2 TxRx/DVB-S2 HDL Receiver/Stream Recovery/BB Decoder/Extract Data Field/Indicate SYNCD bit ==
  rst : Inport  OutDataTypeStr=boolean  PortDimensions=1  SampleTime=7.8125e-09
  Distance : Inport  Port=2  OutDataTypeStr=uint16  PortDimensions=1  SampleTime=7.8125e-09
  validIn : Inport  Port=3  OutDataTypeStr=boolean  PortDimensions=1  SampleTime=7.8125e-09
  Constant1 : Constant  OutDataTypeStr=fixdt(0,1,0)  SampleTime=-1
  Constant2 : Constant  Value=0  OutDataTypeStr=fixdt(0,1,0)  SampleTime=-1
  HDL Counter1 : hdlsllib/Sources/HDL Counter  CountType=Free running  CountInit=0  CountStep=1  CountMax=25  CountFromType=Initial value  CountFrom=0  CountResetPort=on  CountLoadPort=off  CountEnbPort=on  CountDirPort=off  CountHitOutputPort=off  CountDataType=Unsigned  CountWordLen=16  CountFracLen=0  CountSampTime=1
  Logical Operator3 : Logic  AllPortsSameDT=off  OutDataTypeStr=boolean
  Relational Operator1 : RelationalOperator  Operator===  OutDataTypeStr=boolean  RndMeth=Simplest  InputSameDT=off
  Subtract1 : Sum  Inputs=+-  OutDataTypeStr=uint16
  Switch : Switch  Criteria=u2 ~= 0  OutDataTypeStr=fixdt(0, 1, 0)  SaturateOnIntegerOverflow=off  InputSameDT=off
  trigger : Outport  SampleTime=7.8125e-09
  wires:
  HDL Counter1/1 -> Relational Operator1/2
  Constant2/1 -> Switch/3
  Constant1/1 -> Switch/1
  Distance/1 -> Subtract1/1, Switch/2
  Switch/1 -> Subtract1/2
  validIn/1 -> Logical Operator3/2, HDL Counter1/2
  rst/1 -> HDL Counter1/1
  Subtract1/1 -> Relational Operator1/1
  Relational Operator1/1 -> Logical Operator3/1
  Logical Operator3/1 -> trigger/1

== system gm_soc_dvbs2_fpga/DVBS2/DVBS2 TxRx/DVB-S2 HDL Receiver/Stream Recovery/BB Decoder/Extract Data Field/Sample Discard Control ==
  dataIn : Inport  OutDataTypeStr=boolean  PortDimensions=1  SampleTime=7.8125e-09
  startIn : Inport  Port=2  OutDataTypeStr=boolean  PortDimensions=1  SampleTime=7.8125e-09
  endIn : Inport  Port=3  OutDataTypeStr=boolean  PortDimensions=1  SampleTime=7.8125e-09
  validIn : Inport  Port=4  OutDataTypeStr=boolean  PortDimensions=1  SampleTime=7.8125e-09
  Sample Discard Control : MATLAB Function  TreatAsAtomicUnit=on
  dataOut : Outport  SampleTime=7.8125e-09
  startOut : Outport  Port=2  SampleTime=7.8125e-09
  endOut : Outport  Port=3  SampleTime=7.8125e-09
  validOut : Outport  Port=4  SampleTime=7.8125e-09
  wires:
  endIn/1 -> Sample Discard Control/3(endIn)
  dataIn/1 -> Sample Discard Control/1(dataIn)
  validIn/1 -> Sample Discard Control/4(validIn)
  startIn/1 -> Sample Discard Control/2(startIn)
  Sample Discard Control/3(endOut) -> endOut/1
  Sample Discard Control/1(dataOut) -> dataOut/1
  Sample Discard Control/4(validOut) -> validOut/1
  Sample Discard Control/2(startOut) -> startOut/1

== system gm_soc_dvbs2_fpga/DVBS2/DVBS2 TxRx/DVB-S2 HDL Receiver/Stream Recovery/BB Decoder/Extract Stream/Extract User Packet  ==
  SYNCD : Inport  OutDataTypeStr=uint16  PortDimensions=1  SampleTime=7.8125e-09
  bitsIn : Inport  Port=2  OutDataTypeStr=boolean  PortDimensions=1  SampleTime=7.8125e-09
  startIn : Inport  Port=3  OutDataTypeStr=boolean  PortDimensions=1  SampleTime=7.8125e-09
  endIn : Inport  Port=4  OutDataTypeStr=boolean  PortDimensions=1  SampleTime=7.8125e-09
  validIn : Inport  Port=5  OutDataTypeStr=boolean  PortDimensions=1  SampleTime=7.8125e-09
  UPL : Inport  Port=6  OutDataTypeStr=uint16  PortDimensions=1  SampleTime=7.8125e-09
  Compare To Constant : simulink/Logic and Bit Operations/Compare To Constant  relop=~=  const="fi(0,0,16,0,\"hex\",\"0000\")"  OutDataTypeStr=boolean
  Delay{1..2,4..7,9..10,12,19,21} (11 alike) : Delay  DelayLength=double(1)  InitialCondition=0  SampleTime=7.8125e-09
  Indicate SYNCD bit : Subsystem
  Logical Operator : Logic  AllPortsSameDT=off  OutDataTypeStr=boolean  SampleTime=7.8125e-09
  Logical Operator1 : Logic  AllPortsSameDT=off  OutDataTypeStr=boolean  SampleTime=7.8125e-09
  Logical Operator2 : Logic  Operator=NOT  Inputs=1  AllPortsSameDT=off  OutDataTypeStr=boolean  SampleTime=7.8125e-09
  Logical Operator3 : Logic  Operator=OR  AllPortsSameDT=off  OutDataTypeStr=boolean  SampleTime=7.8125e-09
  Sample Discard Control : Subsystem
  Sample Discard Control_term1 : Terminator
  Variable Count Limited HDL Counter : Subsystem
  t : Demux  Outputs=2
  dataOut : Outport  SampleTime=7.8125e-09
  startOut : Outport  Port=2  SampleTime=7.8125e-09
  endOut : Outport  Port=3  SampleTime=7.8125e-09
  validOut : Outport  Port=4  SampleTime=7.8125e-09
  invalidPkt : Outport  Port=5  SampleTime=7.8125e-09
  wires:
  bitsIn/1 -> Delay19/1
  Delay6/1 -> Variable Count Limited HDL Counter/2(countToValue)
  endIn/1 -> Delay7/1
  Delay4/1 -> Delay10/1
  Delay2/1 -> Delay5/1, Indicate SYNCD bit/3(validIn)
  UPL/1 -> Compare To Constant/1, Delay21/1
  Delay5/1 -> Sample Discard Control/4(validIn), Variable Count Limited HDL Counter/3(enb)
  Indicate SYNCD bit/1(trigger) -> Delay12/1, Variable Count Limited HDL Counter/1(rst)
  validIn/1 -> Logical Operator/2
  Delay7/1 -> Delay9/1
  startIn/1 -> Indicate SYNCD bit/1(rst)
  Delay10/1 -> dataOut/1
  Compare To Constant/1 -> Logical Operator/1
  Delay21/1 -> Delay6/1
  Delay19/1 -> Delay4/1
  SYNCD/1 -> Delay1/1
  Logical Operator/1 -> Delay2/1
  Delay1/1 -> Indicate SYNCD bit/2(Distance)
  Variable Count Limited HDL Counter/1(Hit) -> Sample Discard Control/1(dataIn)
  Delay12/1 -> Sample Discard Control/2(startIn)
  Delay9/1 -> Sample Discard Control/3(endIn)
  Sample Discard Control/1(dataOut) -> t/1
  Sample Discard Control/2(startOut) -> Sample Discard Control_term1/1
  Sample Discard Control/3(endOut) -> Logical Operator1/2, Logical Operator3/2
  Sample Discard Control/4(validOut) -> validOut/1
  Logical Operator3/1 -> endOut/1
  t/1 -> startOut/1
  t/2 -> Logical Operator3/1, Logical Operator2/1
  Logical Operator2/1 -> Logical Operator1/1
  Logical Operator1/1 -> invalidPkt/1
